simulink model "ioled"  (Simulink 6.0)
settings: Solver=ode5  StartTime=0.0  StopTime=10  RelTol=1e-3
libraries: xpclib x1
settings Model: Creator=ekbas  LastModifiedBy=ekbas  ExtModeArmWhenConnect=off  BufferReuse=off
settings ConfigSet: SimulationMode=external
settings DataIOCC: SignalLoggingName=sigsOut
settings OptimizationCC: InlineInvariantSignals=off  OptimizeBlockIOStorage=off  BufferReuse=off  LocalBlockOutputs=off
settings DebuggingCC: CheckExecutionContextPreStartOutputMsg=on  CheckExecutionContextRuntimeOutputMsg=on  SolverPrmCheckMsg=none
settings RTWCC: SystemTargetFile=xpctarget.tlc  TemplateMakefile=xpc_default_tmf  ProcessScript=xpctarget_make_rtw_hook
settings xpcTargetCC: TargetFcnLib=ansi_tfl_tmw.mat  GenFloatMathFcnCalls=ANSI_C  ModelReferenceCompliant=off  LifeSpan=inf
settings SFSimCC: SFSimApplyToAllLibs=on  SFSimBuildMode=Incremental

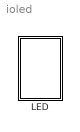
== system ioled ==
  LED : Subsystem  PropExecContextAcrossSSBoundary=on

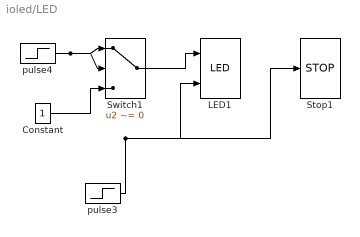
== system ioled/LED ==
  Constant : Constant
  LED1 : xpclib/LED/MathWorks/LED   leds=[1 2]  reset=[0]  initValue=[0]  sampleTime=0.001
  Stop1 : Stop
  Switch1 : Switch  Criteria=u2 ~= 0  SaturateOnIntegerOverflow=on
  pulse3 : Step  Time=4  SampleTime=0
  pulse4 : Step  Time=4  Before=1  After=0  SampleTime=0
  wires:
  pulse3/1 -> Stop1/1, LED1/2
  pulse4/1 -> Switch1/1, Switch1/2
  Switch1/1 -> LED1/1
  Constant/1 -> Switch1/3
